simulink model "buck_converter_DE_Parallel"  (R2023b)
settings: Solver=VariableStepAuto  StartTime=0.0  StopTime=Tend  RelTol=1e-3
values from neighbouring files (symbols this model uses):
  Cdc = 1e-4    (= 0.0001)    [main.m]    (also in main_DE_Parallel.m)
  Ki = Ki_best    [main.m]    (also in main_DE_Parallel.m)
  Kp = Kp_best    [main.m]    (also in main_DE_Parallel.m)
  L = 1e-4    (= 0.0001)    [main.m]    (also in main_DE_Parallel.m = DE_out.best_sol(1,3,end))
  Ro = 1    [main.m]    (also in main_DE_Parallel.m)
  Ts = 1/Fs    (= 0.0001)    [main.m]    (also in main_DE_Parallel.m)
  Tsamp = 1/Fsamp    (= 1e-06)    [main.m]    (also in main_DE_Parallel.m)
  Ttrig = Tend/2    (= 0.05)    [main.m]    (also in main_DE_Parallel.m)
  Vg = 100    [main.m]    (also in main_DE_Parallel.m)
  Vref1 = 40    [main.m]    (also in main_DE_Parallel.m)
  Vref2 = 60    [main.m]    (also in main_DE_Parallel.m)
libraries: spsSeriesRLCBranchLib x3, spsBuckConverterLib x1, spsCurrentMeasurementLib x1, spsDCVoltageSourceLib x1, spsVoltageMeasurementLib x1, simulink x1, simulink_extras x1, sps_lib x1
settings Model: Creator=baik3-ad  LastModifiedBy=baikhyeongmeon

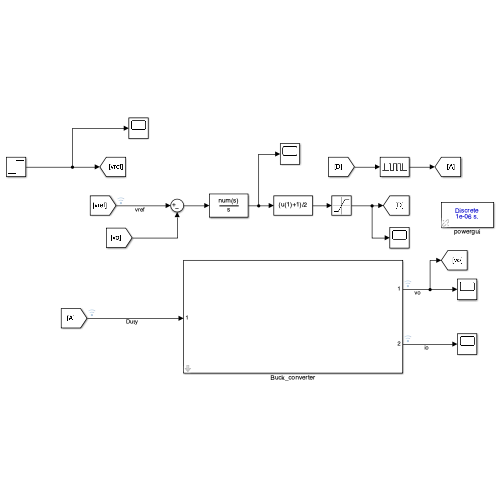
[thumbnail: Simulink's stored preview of the top-level diagram]
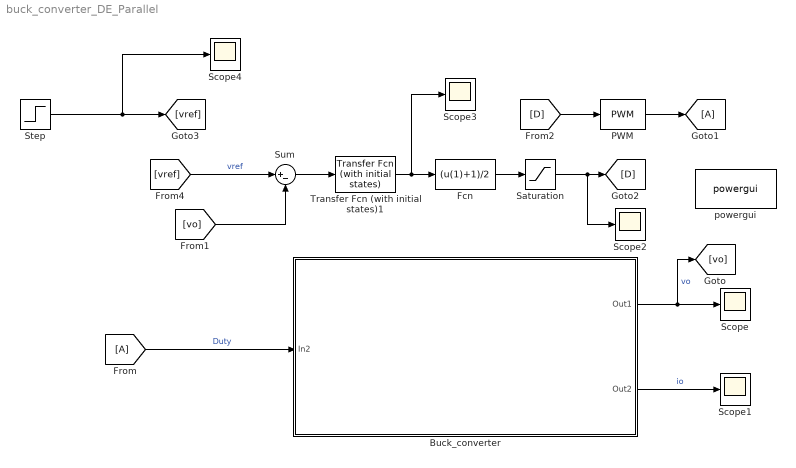
== system buck_converter_DE_Parallel ==
  Buck_converter : Subsystem  mask{Vg=Vg, L=L, C=Cdc, R=Ro}
      mask prompts: Vg "Input voltage"; L "Output inductor"; C "Output capacitor"; R "Output resistor"
  Fcn : Fcn  Expr=(u(1)+1)/2
  From : From
  Goto1 : Goto
  PWM : simulink/Discontinuities/PWM  DisableCoverage=on  Period=Ts  InitialDelay=0  DisallowZeroDutyCycle=off  RunAtFixedTimeIntervals=off  SampleTime=0.1
  Saturation : Saturate  UpperLimit=1  LowerLimit=0
  Scope{,1..4} (5 alike) : Scope
  Step : Step  Time=Ttrig  Before=Vref1  After=Vref2  SampleTime=Tsamp
  Sum : Sum  Inputs=|+-
  Transfer Fcn (with initial states)1 : simulink_extras/Additional Linear/Transfer Fcn (with initial states)  N=[Kp Ki]  D="[1  0]"  X0=0
  powergui : sps_lib/powergui  Priority=1  SimulationMode=Discrete  SampleTime=Tsamp  frequency=60  Iterations=50  frequencyindice=0  Pbase=100e6  ErrMax=1e-4  UnitsV=kV  UnitsW=MW  buscounter=0  FunctionMessages=off  echomessages=off  EnableUseOfTLC=off  CurrentSourceSwitches=off  DisableSnubberDevices=off  DisableRonSwitches=off  DisableVfSwitches=off  DisplayEquations=off  AutomaticDiscreteSolvers=off  SolverType=Tustin/Backward Euler (TBE)  Interpol=off  ExternalGateDelay=off  methode=off  Ts=100  x0status=blocks  SPID=on  SwTol=0  HookPort=off  NonlinearTolerance=1e-4  nMaxIteration=100  ContinueOnMaxIteration=off  RestoreLinks=warning  ResistiveCurrentMeasurement=off  Frange=[0:2:500]  Ylog=off  Xlog=on  ShowGrid=off  save=off  variable=ZData  structure=0  ZoomFFT=off  StartTime=0.0  cycles=1  DisplayStyle=1  fundamental=60  FreqAxis=off  MaxFrequency=1000  frequencyindicesteady=1  RmsSteady=1  display=off
  wires:
  From/1 -> Buck_converter/1(In2)  "Duty"
  Buck_converter/1(Out1) -> [vo], Scope/1  "vo"
  Buck_converter/2(Out2) -> Scope1/1  "io"
  [vref] -> Sum/1  "vref"
  Fcn/1 -> Saturation/1
  Sum/1 -> Transfer Fcn (with initial states)1/1
  Step/1 -> Scope4/1, [vref]
  Saturation/1 -> Scope2/1, [D]
  Transfer Fcn (with initial states)1/1 -> Scope3/1, Fcn/1
  [vo] -> Sum/2
  [D] -> PWM/1
  PWM/1 -> Goto1/1

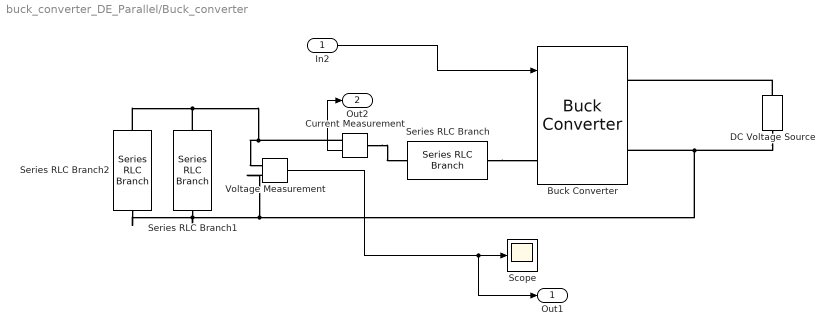
== system buck_converter_DE_Parallel/Buck_converter ==
  In2 : Inport
  Buck Converter : spsBuckConverterLib/Buck Converter  ModelType=Switching devices  Ron=1e-3  Rs=1e6  Cs=inf  Vforward=[0,0]  Ron_Diode=1e-3  Rs_Diode=1e6  Cs_Diode=inf  Vf_Diode=1e-3  Rs_CurrentSource=inf  Ron_ACsource=1e-3
      settings: LibrarySourceBlock=sps_lib/Power Electronics/Buck Converter
  Current Measurement : spsCurrentMeasurementLib/Current Measurement  PhasorSimulation=off  OutputType=Complex  PSBequivalent=0
  DC Voltage Source : spsDCVoltageSourceLib/DC Voltage Source  Amplitude=Vg  Measurements=None
  Scope : Scope
  Series RLC Branch : spsSeriesRLCBranchLib/Series RLC Branch  LConnTagsString=__new0  RConnTagsString=__new0  BranchType=L  Resistance=1  Inductance=L  SetiL0=off  InitialCurrent=0  Capacitance=1e-6  Setx0=off  InitialVoltage=0  Measurements=None
  Series RLC Branch1 : spsSeriesRLCBranchLib/Series RLC Branch  LConnTagsString=__new0  RConnTagsString=__new0  BranchType=C  Resistance=1  Inductance=1e-3  SetiL0=off  InitialCurrent=0  Capacitance=C  Setx0=off  InitialVoltage=0  Measurements=None
  Series RLC Branch2 : spsSeriesRLCBranchLib/Series RLC Branch  LConnTagsString=__new0  RConnTagsString=__new0  BranchType=R  Resistance=R  Inductance=1e-3  SetiL0=off  InitialCurrent=0  Capacitance=1e-6  Setx0=off  InitialVoltage=0  Measurements=None
  Voltage Measurement : spsVoltageMeasurementLib/Voltage Measurement  PhasorSimulation=off  OutputType=Complex  PSBequivalent=0
  Out1 : Outport
  Out2 : Outport  Port=2
  wires:
  In2/1 -> Buck Converter/1
  Voltage Measurement/1 -> Out1/1, Scope/1
  Current Measurement/1 -> Out2/1
  connections:
  Voltage Measurement/LConn2 -- Series RLC Branch2/RConn1 -- Series RLC Branch1/RConn1 -- Buck Converter/RConn2 -- DC Voltage Source/LConn1
  Series RLC Branch2/LConn1 -- Series RLC Branch1/LConn1 -- Current Measurement/RConn1 -- Voltage Measurement/LConn1
  DC Voltage Source/RConn1 -- Buck Converter/RConn1
  Series RLC Branch/LConn1 -- Buck Converter/LConn1
  Current Measurement/LConn1 -- Series RLC Branch/RConn1
